simulink model "kin_test"  (R2018b)
settings: Solver=FixedStepAuto  StartTime=0.0  StopTime=100  FixedStep=0.1  RelTol=1e-3
libraries: simulink x2, cstblocks x1
settings Model: Creator=le'e'x'  LastModifiedBy=le'e'x'

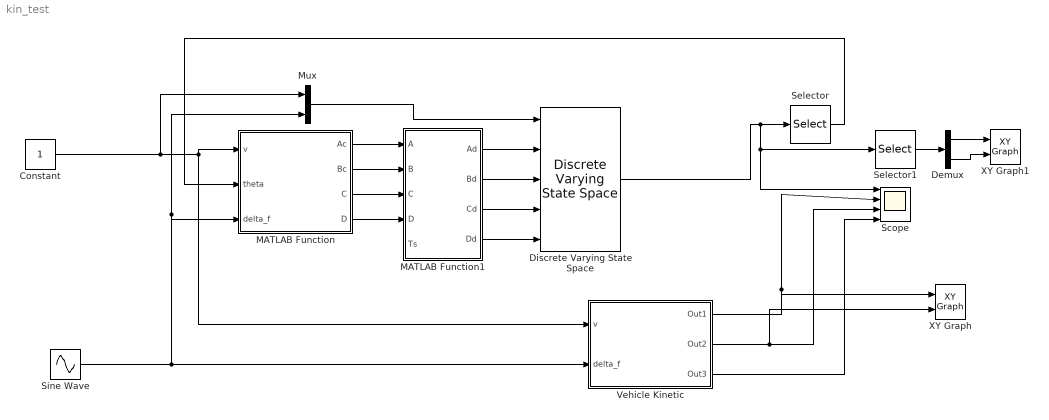
== system kin_test ==
  Constant : Constant
  Demux : Demux  Outputs=2
  Discrete Varying State Space : cstblocks/Linear Parameter Varying/Discrete Varying State Space  x0=0  Ts=-1  OutputX=off  OutputDX=off
      settings: SourceProductName=Control System Toolbox  SourceProductBaseCode=CT
  MATLAB Function : MATLAB Function  TreatAsAtomicUnit=on
  MATLAB Function1 : MATLAB Function  TreatAsAtomicUnit=on
  Mux : Mux  Inputs=2
  Scope : Scope  NumInputPorts=4
  Selector : Selector  InputPortWidth=3  IndexOptions=Index vector (dialog)  Indices=[3]  OutputSizes=1
  Selector1 : Selector  InputPortWidth=3  IndexOptions=Index vector (dialog)  Indices=[1 2]  OutputSizes=1
  Sine Wave : Sin  Amplitude=0  Bias=deg2rad(30)  SampleTime=0
  Vehicle Kinetic : Subsystem  AncestorBlock=my_library/Vehicle Kinetic  mask{x=0, y=0, fai=0, L=2.6}
      mask prompts: x "X_0"; y "Y_0"; fai "Phi_0"
      mask Display:
      | port_label('input',1,'v','texmode','on')
      | port_label('input',2,'\delta_f','texmode','on')
      | port_label('output',1,'x','texmode','on')
      | port_label('output',2,'y','texmode','on')
      | port_label('output',3,'\phi','texmode','on')
      | disp("Vehicle Kinetic")
  XY Graph : simulink/Sinks/XY Graph  xmin=-100  xmax=100  ymin=-100  ymax=100  st=-1
  XY Graph1 : simulink/Sinks/XY Graph  xmin=-100  xmax=100  ymin=-100  ymax=100  st=-1
  wires:
  Constant/1 -> Mux/1, Vehicle Kinetic/1(v), MATLAB Function/1(v)
  Sine Wave/1 -> Vehicle Kinetic/2(delta_f), Mux/2, MATLAB Function/3(delta_f)
  Discrete Varying State Space/1 -> Selector1/1, Scope/1, Selector/1
  Selector/1 -> MATLAB Function/2(theta)
  Vehicle Kinetic/1(Out1) -> Scope/2, XY Graph/1
  Vehicle Kinetic/2(Out2) -> XY Graph/2, Scope/3
  Vehicle Kinetic/3(Out3) -> Scope/4
  Selector1/1 -> Demux/1
  Demux/1 -> XY Graph1/1
  Demux/2 -> XY Graph1/2
  MATLAB Function/1(Ac) -> MATLAB Function1/1(A)
  MATLAB Function/2(Bc) -> MATLAB Function1/2(B)
  MATLAB Function/3(C) -> MATLAB Function1/3(C)
  MATLAB Function/4(D) -> MATLAB Function1/4(D)
  MATLAB Function1/4(Dd) -> Discrete Varying State Space/5
  MATLAB Function1/3(Cd) -> Discrete Varying State Space/4
  MATLAB Function1/2(Bd) -> Discrete Varying State Space/3
  MATLAB Function1/1(Ad) -> Discrete Varying State Space/2
  Mux/1 -> Discrete Varying State Space/1

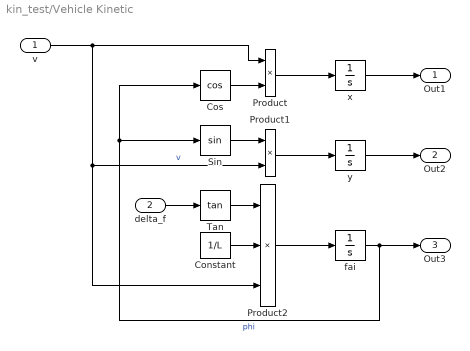
== system kin_test/Vehicle Kinetic ==
  v : Inport
  delta_f : Inport  Port=2
  Constant : Constant  Value=1/L
  Cos : Trigonometry  Operator=cos
  Product : Product
  Product1 : Product
  Product2 : Product  Inputs=3
  Sin : Trigonometry
  Tan : Trigonometry  Operator=tan
  fai : Integrator  InitialCondition=fai
  x : Integrator  InitialCondition=x
  y : Integrator  InitialCondition=y
  Out1 : Outport
  Out2 : Outport  Port=2
  Out3 : Outport  Port=3
  wires:
  x/1 -> Out1/1
  fai/1 -> Out3/1, Sin/1, Cos/1  "phi"
  Cos/1 -> Product/2
  v/1 -> Product2/3, Product1/2, Product/1  "v"
  Product/1 -> x/1
  Sin/1 -> Product1/1
  Product1/1 -> y/1
  y/1 -> Out2/1
  Tan/1 -> Product2/1
  Constant/1 -> Product2/2
  delta_f/1 -> Tan/1
  Product2/1 -> fai/1

== matlab function kin_test/MATLAB Function1 ==
  data: A input; Ad output; B input; C input; D input; Ts input; Bd output; Cd output; Dd output
function [Ad,Bd,Cd,Dd] = fcn(A,B,C,D,Ts)
%#codegen
Cd=C;
Dd=D;
Ad=(eye(size(A))+Ts*A/2)/(eye(size(A))-Ts*A/2);
Bd=Ts*B;

== matlab function kin_test/MATLAB Function ==
  data: v input; Ac output; theta input; delta_f input; Bc output; C output; D output
function [Ac,Bc,C,D] = fcn(v,theta,delta_f)
%#codegen
L=2.6;
Ac=[ 0, 0, -v*sin(theta);
    0, 0,  v*cos(theta);
    0, 0,             0];
Bc =[  cos(theta),                      0;
    sin(theta),                      0;
    tan(delta_f)/L, (v*(tan(delta_f)^2 + 1))/L];
C=eye(3,3);
D=zeros(3,2);
